simulink model "dspace_2019"  (R2019b)
settings: Solver=FixedStepDiscrete  StartTime=0.0  StopTime=Inf  FixedStep=1e-3  RelTol=1e-3
PostLoadFcn:
  | , if any(exist('dsrtsu_mdlpostloadfcn', 'file') ~= 0), dsrtsu_mdlpostloadfcn('Execute', bdroot); end,
undefined symbols (not defined in the file): ami, amk1_setpoints_1, amk2_setpoints_1, amk3_setpoints_1, amk4_setpoints_1, as, digital, ebs, indicator, mcu_set_dbu_indicator_points, mcu_set_ecu_indicator_points, res_ntm_node_control
libraries: rtican x63, simulink x5, rti1401lib_dio_type3 x4, simulink_extras x1
(part 16 of 16)

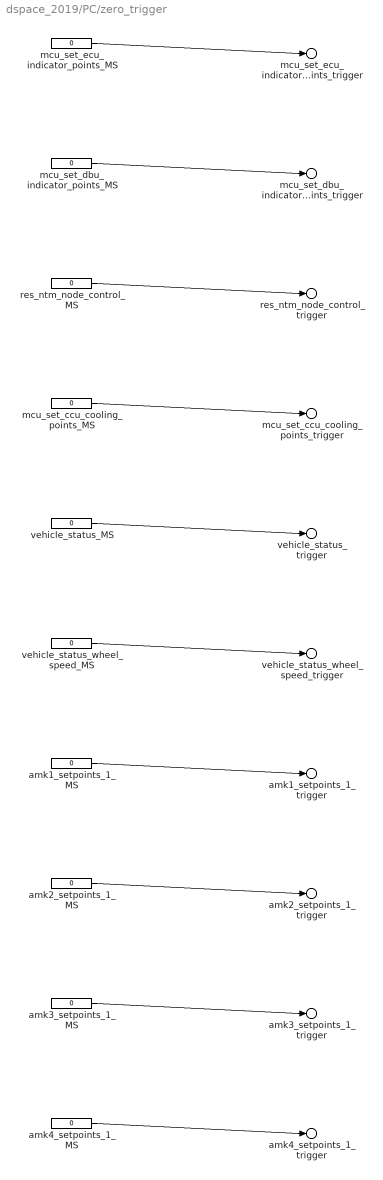
== system dspace_2019/PC/zero_trigger ==
  amk1_setpoints_1_MS : Constant  Value=0
  amk2_setpoints_1_MS : Constant  Value=0
  amk3_setpoints_1_MS : Constant  Value=0
  amk4_setpoints_1_MS : Constant  Value=0
  mcu_set_ccu_cooling_points_MS : Constant  Value=0
  mcu_set_dbu_indicator_points_MS : Constant  Value=0
  mcu_set_ecu_indicator_points_MS : Constant  Value=0
  res_ntm_node_control_MS : Constant  Value=0
  vehicle_status_MS : Constant  Value=0
  vehicle_status_wheel_speed_MS : Constant  Value=0
  mcu_set_ecu_indicator_points_trigger : Outport  PortName=triggers  Element=mcu_set_ecu_indicator_points
  mcu_set_dbu_indicator_points_trigger : Outport  PortName=triggers  Element=mcu_set_dbu_indicator_points
  res_ntm_node_control_trigger : Outport  PortName=triggers  Element=res_ntm_node_control
  mcu_set_ccu_cooling_points_trigger : Outport  PortName=triggers  Element=mcu_set_ccu_cooling_points
  vehicle_status_trigger : Outport  PortName=triggers  Element=vehicle_status
  vehicle_status_wheel_speed_trigger : Outport  PortName=triggers  Element=vehicle_status_wheel_speed
  amk1_setpoints_1_trigger : Outport  PortName=triggers  Element=amk1_setpoints_1
  amk2_setpoints_1_trigger : Outport  PortName=triggers  Element=amk2_setpoints_1
  amk3_setpoints_1_trigger : Outport  PortName=triggers  Element=amk3_setpoints_1
  amk4_setpoints_1_trigger : Outport  PortName=triggers  Element=amk4_setpoints_1
  wires:
  mcu_set_ecu_indicator_points_MS/1 -> mcu_set_ecu_indicator_points_trigger/1
  mcu_set_dbu_indicator_points_MS/1 -> mcu_set_dbu_indicator_points_trigger/1
  res_ntm_node_control_MS/1 -> res_ntm_node_control_trigger/1
  mcu_set_ccu_cooling_points_MS/1 -> mcu_set_ccu_cooling_points_trigger/1
  vehicle_status_MS/1 -> vehicle_status_trigger/1
  vehicle_status_wheel_speed_MS/1 -> vehicle_status_wheel_speed_trigger/1
  amk1_setpoints_1_MS/1 -> amk1_setpoints_1_trigger/1
  amk2_setpoints_1_MS/1 -> amk2_setpoints_1_trigger/1
  amk3_setpoints_1_MS/1 -> amk3_setpoints_1_trigger/1
  amk4_setpoints_1_MS/1 -> amk4_setpoints_1_trigger/1

== system dspace_2019/PC/zero_tx  ==
  inner : Subsystem
  mcu_set_ecu_indicator_points_outbus : Outport  PortName=signals  Element=mcu_set_ecu_indicator_points
  mcu_set_dbu_indicator_points_outbus : Outport  PortName=signals  Element=mcu_set_dbu_indicator_points
  res_ntm_node_control_outbus : Outport  PortName=signals  Element=res_ntm_node_control
  mcu_set_ccu_cooling_points_outbus : Outport  PortName=signals  Element=mcu_set_ccu_cooling_points
  vehicle_status_outbus : Outport  PortName=signals  Element=vehicle_status
  vehicle_status_wheel_speed_outbus : Outport  PortName=signals  Element=vehicle_status_wheel_speed
  amk1_setpoints_1_outbus : Outport  PortName=signals  Element=amk1_setpoints_1
  amk2_setpoints_1_outbus : Outport  PortName=signals  Element=amk2_setpoints_1
  amk3_setpoints_1_outbus : Outport  PortName=signals  Element=amk3_setpoints_1
  amk4_setpoints_1_outbus : Outport  PortName=signals  Element=amk4_setpoints_1
  wires:
  inner/10(mcu_set_ecu_indicator_points) -> mcu_set_ecu_indicator_points_outbus/1
  inner/9(mcu_set_dbu_indicator_points) -> mcu_set_dbu_indicator_points_outbus/1
  inner/8(res_ntm_node_control) -> res_ntm_node_control_outbus/1
  inner/7(mcu_set_ccu_cooling_points) -> mcu_set_ccu_cooling_points_outbus/1
  inner/6(vehicle_status) -> vehicle_status_outbus/1
  inner/5(vehicle_status_wheel_speed) -> vehicle_status_wheel_speed_outbus/1
  inner/4(amk1_setpoints_1) -> amk1_setpoints_1_outbus/1
  inner/3(amk2_setpoints_1) -> amk2_setpoints_1_outbus/1
  inner/2(amk3_setpoints_1) -> amk3_setpoints_1_outbus/1
  inner/1(amk4_setpoints_1) -> amk4_setpoints_1_outbus/1

== system dspace_2019/RTI Data/RTI Data Store ==
  RTI Data Store : Subsystem  mask(RTI_DATA_STORE){}
      mask help:
      | RTI Data Store Block. This block is used by RTI to store internal model dependent data. Deleting this block will result in data loss.
      |
      | NEVER DELETE, COPY, OR MODIFY THIS BLOCK!
      mask Help:
      | RTI Data Store Block. This block is used by RTI to store internal model dependent data. Deleting this block will result in data loss.
      | 
      | NEVER DELETE, COPY, OR MODIFY THIS BLOCK!
      mask Display: text(0.5, 0.5, ' ', 'HorizontalAlignment', 'center');

== system dspace_2019/PC/plausability_check/implausability_logic ==
  apps1 : Inport
  apps2 : Inport  Port=2
  Compare To Constant : simulink/Logic and Bit Operations/Compare To Constant  relop=>  const=0.1  OutDataTypeStr=boolean
  Integrator : Integrator  ExternalReset=falling
  MATLAB Function2 : MATLAB Function  TreatAsAtomicUnit=on
  implausability : Outport
  wires:
  apps2/1 -> MATLAB Function2/2(apps2)
  apps1/1 -> MATLAB Function2/1(apps1)
  Compare To Constant/1 -> implausability/1
  MATLAB Function2/1(implausability) -> Integrator/2, Integrator/1
  Integrator/1 -> Compare To Constant/1

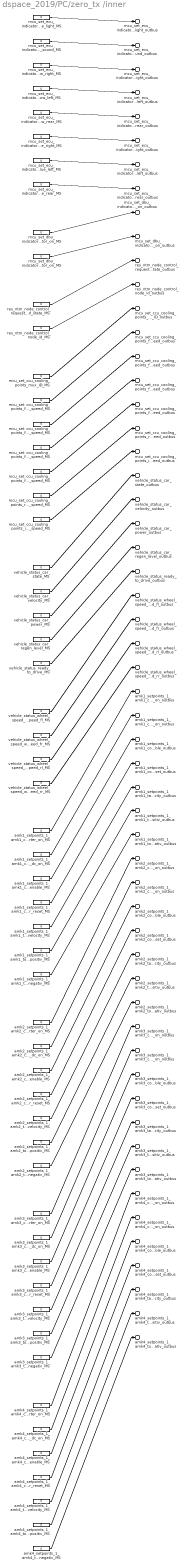
== system dspace_2019/PC/zero_tx /inner ==
  amk1_setpoints_1_amk1_control_dc_on_MS : Constant  Value=0
  amk1_setpoints_1_amk1_control_enable_MS : Constant  Value=0
  amk1_setpoints_1_amk1_control_error_reset_MS : Constant  Value=0
  amk1_setpoints_1_amk1_control_inverter_on_MS : Constant  Value=0
  amk1_setpoints_1_amk1_target_velocity_MS : Constant  Value=0
  amk1_setpoints_1_amk1_torque_limit_negativ_MS : Constant  Value=0
  amk1_setpoints_1_amk1_torque_limit_positiv_MS : Constant  Value=0
  amk2_setpoints_1_amk2_control_dc_on_MS : Constant  Value=0
  amk2_setpoints_1_amk2_control_enable_MS : Constant  Value=0
  amk2_setpoints_1_amk2_control_error_reset_MS : Constant  Value=0
  amk2_setpoints_1_amk2_control_inverter_on_MS : Constant  Value=0
  amk2_setpoints_1_amk2_target_velocity_MS : Constant  Value=0
  amk2_setpoints_1_amk2_torque_limit_negativ_MS : Constant  Value=0
  amk2_setpoints_1_amk2_torque_limit_positiv_MS : Constant  Value=0
  amk3_setpoints_1_amk3_control_dc_on_MS : Constant  Value=0
  amk3_setpoints_1_amk3_control_enable_MS : Constant  Value=0
  amk3_setpoints_1_amk3_control_error_reset_MS : Constant  Value=0
  amk3_setpoints_1_amk3_control_inverter_on_MS : Constant  Value=0
  amk3_setpoints_1_amk3_target_velocity_MS : Constant  Value=0
  amk3_setpoints_1_amk3_torque_limit_negativ_MS : Constant  Value=0
  amk3_setpoints_1_amk3_torque_limit_positiv_MS : Constant  Value=0
  amk4_setpoints_1_amk4_control_dc_on_MS : Constant  Value=0
  amk4_setpoints_1_amk4_control_enable_MS : Constant  Value=0
  amk4_setpoints_1_amk4_control_error_reset_MS : Constant  Value=0
  amk4_setpoints_1_amk4_control_inverter_on_MS : Constant  Value=0
  amk4_setpoints_1_amk4_target_velocity_MS : Constant  Value=0
  amk4_setpoints_1_amk4_torque_limit_negativ_MS : Constant  Value=0
  amk4_setpoints_1_amk4_torque_limit_positiv_MS : Constant  Value=0
  mcu_set_ccu_cooling_points_fan1_speed_MS : Constant  Value=0
  mcu_set_ccu_cooling_points_fan2_speed_MS : Constant  Value=0
  mcu_set_ccu_cooling_points_fan3_speed_MS : Constant  Value=0
  mcu_set_ccu_cooling_points_fron_pump_speed_MS : Constant  Value=0
  mcu_set_ccu_cooling_points_inverter_pump_speed_MS : Constant  Value=0
  mcu_set_ccu_cooling_points_mux_ID_MS : Constant  Value=0
  mcu_set_ccu_cooling_points_rear_pump_speed_MS : Constant  Value=0
  mcu_set_dbu_indicator_points_r2d_indicator_on_MS : Constant  Value=0
  mcu_set_dbu_indicator_points_ts_indicator_on_MS : Constant  Value=0
  mcu_set_ecu_indicator_points_assi_blue_left_MS : Constant  Value=0
  mcu_set_ecu_indicator_points_assi_blue_rear_MS : Constant  Value=0
  mcu_set_ecu_indicator_points_assi_blue_right_MS : Constant  Value=0
  mcu_set_ecu_indicator_points_assi_yellow_left_MS : Constant  Value=0
  mcu_set_ecu_indicator_points_assi_yellow_rear_MS : Constant  Value=0
  mcu_set_ecu_indicator_points_assi_yellow_right_MS : Constant  Value=0
  mcu_set_ecu_indicator_points_brake_light_MS : Constant  Value=0
  mcu_set_ecu_indicator_points_r2d_sound_MS : Constant  Value=0
  res_ntm_node_control_node_id_MS : Constant  Value=0
  res_ntm_node_control_requested_state_MS : Constant  Value=0
  vehicle_status_car_power_MS : Constant  Value=0
  vehicle_status_car_regen_level_MS : Constant  Value=0
  vehicle_status_car_state_MS : Constant  Value=0
  vehicle_status_car_velocity_MS : Constant  Value=0
  vehicle_status_ready_to_drive_MS : Constant  Value=0
  vehicle_status_wheel_speed_wheel_speed_fl_MS : Constant  Value=0
  vehicle_status_wheel_speed_wheel_speed_fr_MS : Constant  Value=0
  vehicle_status_wheel_speed_wheel_speed_rl_MS : Constant  Value=0
  vehicle_status_wheel_speed_wheel_speed_rr_MS : Constant  Value=0
  amk4_setpoints_1_amk4_control_inverter_on_outbus : Outport  PortName=amk4_setpoints_1  Element=amk4_control_inverter_on
  amk4_setpoints_1_amk4_control_dc_on_outbus : Outport  PortName=amk4_setpoints_1  Element=amk4_control_dc_on
  amk4_setpoints_1_amk4_control_enable_outbus : Outport  PortName=amk4_setpoints_1  Element=amk4_control_enable
  amk4_setpoints_1_amk4_control_error_reset_outbus : Outport  PortName=amk4_setpoints_1  Element=amk4_control_error_reset
  amk4_setpoints_1_amk4_target_velocity_outbus : Outport  PortName=amk4_setpoints_1  Element=amk4_target_velocity
  amk4_setpoints_1_amk4_torque_limit_positiv_outbus : Outport  PortName=amk4_setpoints_1  Element=amk4_torque_limit_positiv
  amk4_setpoints_1_amk4_torque_limit_negativ_outbus : Outport  PortName=amk4_setpoints_1  Element=amk4_torque_limit_negativ
  amk3_setpoints_1_amk3_control_inverter_on_outbus : Outport  Port=2  PortName=amk3_setpoints_1  Element=amk3_control_inverter_on
  amk3_setpoints_1_amk3_control_dc_on_outbus : Outport  Port=2  PortName=amk3_setpoints_1  Element=amk3_control_dc_on
  amk3_setpoints_1_amk3_control_enable_outbus : Outport  Port=2  PortName=amk3_setpoints_1  Element=amk3_control_enable
  amk3_setpoints_1_amk3_control_error_reset_outbus : Outport  Port=2  PortName=amk3_setpoints_1  Element=amk3_control_error_reset
  amk3_setpoints_1_amk3_target_velocity_outbus : Outport  Port=2  PortName=amk3_setpoints_1  Element=amk3_target_velocity
  amk3_setpoints_1_amk3_torque_limit_positiv_outbus : Outport  Port=2  PortName=amk3_setpoints_1  Element=amk3_torque_limit_positiv
  amk3_setpoints_1_amk3_torque_limit_negativ_outbus : Outport  Port=2  PortName=amk3_setpoints_1  Element=amk3_torque_limit_negativ
  amk2_setpoints_1_amk2_control_inverter_on_outbus : Outport  Port=3  PortName=amk2_setpoints_1  Element=amk2_control_inverter_on
  amk2_setpoints_1_amk2_control_dc_on_outbus : Outport  Port=3  PortName=amk2_setpoints_1  Element=amk2_control_dc_on
  amk2_setpoints_1_amk2_control_enable_outbus : Outport  Port=3  PortName=amk2_setpoints_1  Element=amk2_control_enable
  amk2_setpoints_1_amk2_control_error_reset_outbus : Outport  Port=3  PortName=amk2_setpoints_1  Element=amk2_control_error_reset
  amk2_setpoints_1_amk2_target_velocity_outbus : Outport  Port=3  PortName=amk2_setpoints_1  Element=amk2_target_velocity
  amk2_setpoints_1_amk2_torque_limit_positiv_outbus : Outport  Port=3  PortName=amk2_setpoints_1  Element=amk2_torque_limit_positiv
  amk2_setpoints_1_amk2_torque_limit_negativ_outbus : Outport  Port=3  PortName=amk2_setpoints_1  Element=amk2_torque_limit_negativ
  amk1_setpoints_1_amk1_control_inverter_on_outbus : Outport  Port=4  PortName=amk1_setpoints_1  Element=amk1_control_inverter_on
  amk1_setpoints_1_amk1_control_dc_on_outbus : Outport  Port=4  PortName=amk1_setpoints_1  Element=amk1_control_dc_on
  amk1_setpoints_1_amk1_control_enable_outbus : Outport  Port=4  PortName=amk1_setpoints_1  Element=amk1_control_enable
  amk1_setpoints_1_amk1_control_error_reset_outbus : Outport  Port=4  PortName=amk1_setpoints_1  Element=amk1_control_error_reset
  amk1_setpoints_1_amk1_target_velocity_outbus : Outport  Port=4  PortName=amk1_setpoints_1  Element=amk1_target_velocity
  amk1_setpoints_1_amk1_torque_limit_positiv_outbus : Outport  Port=4  PortName=amk1_setpoints_1  Element=amk1_torque_limit_positiv
  amk1_setpoints_1_amk1_torque_limit_negativ_outbus : Outport  Port=4  PortName=amk1_setpoints_1  Element=amk1_torque_limit_negativ
  vehicle_status_wheel_speed_wheel_speed_fl_outbus : Outport  Port=5  PortName=vehicle_status_wheel_speed  Element=wheel_speed_fl
  vehicle_status_wheel_speed_wheel_speed_fr_outbus : Outport  Port=5  PortName=vehicle_status_wheel_speed  Element=wheel_speed_fr
  vehicle_status_wheel_speed_wheel_speed_rl_outbus : Outport  Port=5  PortName=vehicle_status_wheel_speed  Element=wheel_speed_rl
  vehicle_status_wheel_speed_wheel_speed_rr_outbus : Outport  Port=5  PortName=vehicle_status_wheel_speed  Element=wheel_speed_rr
  vehicle_status_car_state_outbus : Outport  Port=6  PortName=vehicle_status  Element=car_state
  vehicle_status_car_velocity_outbus : Outport  Port=6  PortName=vehicle_status  Element=car_velocity
  vehicle_status_car_power_outbus : Outport  Port=6  PortName=vehicle_status  Element=car_power
  vehicle_status_car_regen_level_outbus : Outport  Port=6  PortName=vehicle_status  Element=car_regen_level
  vehicle_status_ready_to_drive_outbus : Outport  Port=6  PortName=vehicle_status  Element=ready_to_drive
  mcu_set_ccu_cooling_points_mux_ID_outbus : Outport  Port=7  PortName=mcu_set_ccu_cooling_points  Element=mux_ID
  mcu_set_ccu_cooling_points_fan1_speed_outbus : Outport  Port=7  PortName=mcu_set_ccu_cooling_points  Element=fan1_speed
  mcu_set_ccu_cooling_points_fan2_speed_outbus : Outport  Port=7  PortName=mcu_set_ccu_cooling_points  Element=fan2_speed
  mcu_set_ccu_cooling_points_fan3_speed_outbus : Outport  Port=7  PortName=mcu_set_ccu_cooling_points  Element=fan3_speed
  mcu_set_ccu_cooling_points_fron_pump_speed_outbus : Outport  Port=7  PortName=mcu_set_ccu_cooling_points  Element=fron_pump_speed
  mcu_set_ccu_cooling_points_rear_pump_speed_outbus : Outport  Port=7  PortName=mcu_set_ccu_cooling_points  Element=rear_pump_speed
  mcu_set_ccu_cooling_points_inverter_pump_speed_outbus : Outport  Port=7  PortName=mcu_set_ccu_cooling_points  Element=inverter_pump_speed
  res_ntm_node_control_requested_state_outbus : Outport  Port=8  PortName=res_ntm_node_control  Element=requested_state
  res_ntm_node_control_node_id_outbus : Outport  Port=8  PortName=res_ntm_node_control  Element=node_id
  mcu_set_dbu_indicator_points_ts_indicator_on_outbus : Outport  Port=9  PortName=mcu_set_dbu_indicator_points  Element=ts_indicator_on
  mcu_set_dbu_indicator_points_r2d_indicator_on_outbus : Outport  Port=9  PortName=mcu_set_dbu_indicator_points  Element=r2d_indicator_on
  mcu_set_ecu_indicator_points_brake_light_outbus : Outport  Port=10  PortName=mcu_set_ecu_indicator_points  Element=brake_light
  mcu_set_ecu_indicator_points_r2d_sound_outbus : Outport  Port=10  PortName=mcu_set_ecu_indicator_points  Element=r2d_sound
  mcu_set_ecu_indicator_points_assi_yellow_right_outbus : Outport  Port=10  PortName=mcu_set_ecu_indicator_points  Element=assi_yellow_right
  mcu_set_ecu_indicator_points_assi_yellow_left_outbus : Outport  Port=10  PortName=mcu_set_ecu_indicator_points  Element=assi_yellow_left
  mcu_set_ecu_indicator_points_assi_yellow_rear_outbus : Outport  Port=10  PortName=mcu_set_ecu_indicator_points  Element=assi_yellow_rear
  mcu_set_ecu_indicator_points_assi_blue_right_outbus : Outport  Port=10  PortName=mcu_set_ecu_indicator_points  Element=assi_blue_right
  mcu_set_ecu_indicator_points_assi_blue_left_outbus : Outport  Port=10  PortName=mcu_set_ecu_indicator_points  Element=assi_blue_left
  mcu_set_ecu_indicator_points_assi_blue_rear_outbus : Outport  Port=10  PortName=mcu_set_ecu_indicator_points  Element=assi_blue_rear
  wires:
  mcu_set_ecu_indicator_points_brake_light_MS/1 -> mcu_set_ecu_indicator_points_brake_light_outbus/1
  mcu_set_ecu_indicator_points_r2d_sound_MS/1 -> mcu_set_ecu_indicator_points_r2d_sound_outbus/1
  mcu_set_ecu_indicator_points_assi_yellow_right_MS/1 -> mcu_set_ecu_indicator_points_assi_yellow_right_outbus/1
  mcu_set_ecu_indicator_points_assi_yellow_left_MS/1 -> mcu_set_ecu_indicator_points_assi_yellow_left_outbus/1
  mcu_set_ecu_indicator_points_assi_yellow_rear_MS/1 -> mcu_set_ecu_indicator_points_assi_yellow_rear_outbus/1
  mcu_set_ecu_indicator_points_assi_blue_right_MS/1 -> mcu_set_ecu_indicator_points_assi_blue_right_outbus/1
  mcu_set_ecu_indicator_points_assi_blue_left_MS/1 -> mcu_set_ecu_indicator_points_assi_blue_left_outbus/1
  mcu_set_ecu_indicator_points_assi_blue_rear_MS/1 -> mcu_set_ecu_indicator_points_assi_blue_rear_outbus/1
  mcu_set_dbu_indicator_points_ts_indicator_on_MS/1 -> mcu_set_dbu_indicator_points_ts_indicator_on_outbus/1
  mcu_set_dbu_indicator_points_r2d_indicator_on_MS/1 -> mcu_set_dbu_indicator_points_r2d_indicator_on_outbus/1
  res_ntm_node_control_requested_state_MS/1 -> res_ntm_node_control_requested_state_outbus/1
  res_ntm_node_control_node_id_MS/1 -> res_ntm_node_control_node_id_outbus/1
  mcu_set_ccu_cooling_points_mux_ID_MS/1 -> mcu_set_ccu_cooling_points_mux_ID_outbus/1
  mcu_set_ccu_cooling_points_fan1_speed_MS/1 -> mcu_set_ccu_cooling_points_fan1_speed_outbus/1
  mcu_set_ccu_cooling_points_fan2_speed_MS/1 -> mcu_set_ccu_cooling_points_fan2_speed_outbus/1
  mcu_set_ccu_cooling_points_fan3_speed_MS/1 -> mcu_set_ccu_cooling_points_fan3_speed_outbus/1
  mcu_set_ccu_cooling_points_fron_pump_speed_MS/1 -> mcu_set_ccu_cooling_points_fron_pump_speed_outbus/1
  mcu_set_ccu_cooling_points_rear_pump_speed_MS/1 -> mcu_set_ccu_cooling_points_rear_pump_speed_outbus/1
  mcu_set_ccu_cooling_points_inverter_pump_speed_MS/1 -> mcu_set_ccu_cooling_points_inverter_pump_speed_outbus/1
  vehicle_status_car_state_MS/1 -> vehicle_status_car_state_outbus/1
  vehicle_status_car_velocity_MS/1 -> vehicle_status_car_velocity_outbus/1
  vehicle_status_car_power_MS/1 -> vehicle_status_car_power_outbus/1
  vehicle_status_car_regen_level_MS/1 -> vehicle_status_car_regen_level_outbus/1
  vehicle_status_ready_to_drive_MS/1 -> vehicle_status_ready_to_drive_outbus/1
  vehicle_status_wheel_speed_wheel_speed_fl_MS/1 -> vehicle_status_wheel_speed_wheel_speed_fl_outbus/1
  vehicle_status_wheel_speed_wheel_speed_fr_MS/1 -> vehicle_status_wheel_speed_wheel_speed_fr_outbus/1
  vehicle_status_wheel_speed_wheel_speed_rl_MS/1 -> vehicle_status_wheel_speed_wheel_speed_rl_outbus/1
  vehicle_status_wheel_speed_wheel_speed_rr_MS/1 -> vehicle_status_wheel_speed_wheel_speed_rr_outbus/1
  amk1_setpoints_1_amk1_control_inverter_on_MS/1 -> amk1_setpoints_1_amk1_control_inverter_on_outbus/1
  amk1_setpoints_1_amk1_control_dc_on_MS/1 -> amk1_setpoints_1_amk1_control_dc_on_outbus/1
  amk1_setpoints_1_amk1_control_enable_MS/1 -> amk1_setpoints_1_amk1_control_enable_outbus/1
  amk1_setpoints_1_amk1_control_error_reset_MS/1 -> amk1_setpoints_1_amk1_control_error_reset_outbus/1
  amk1_setpoints_1_amk1_target_velocity_MS/1 -> amk1_setpoints_1_amk1_target_velocity_outbus/1
  amk1_setpoints_1_amk1_torque_limit_positiv_MS/1 -> amk1_setpoints_1_amk1_torque_limit_positiv_outbus/1
  amk1_setpoints_1_amk1_torque_limit_negativ_MS/1 -> amk1_setpoints_1_amk1_torque_limit_negativ_outbus/1
  amk2_setpoints_1_amk2_control_inverter_on_MS/1 -> amk2_setpoints_1_amk2_control_inverter_on_outbus/1
  amk2_setpoints_1_amk2_control_dc_on_MS/1 -> amk2_setpoints_1_amk2_control_dc_on_outbus/1
  amk2_setpoints_1_amk2_control_enable_MS/1 -> amk2_setpoints_1_amk2_control_enable_outbus/1
  amk2_setpoints_1_amk2_control_error_reset_MS/1 -> amk2_setpoints_1_amk2_control_error_reset_outbus/1
  amk2_setpoints_1_amk2_target_velocity_MS/1 -> amk2_setpoints_1_amk2_target_velocity_outbus/1
  amk2_setpoints_1_amk2_torque_limit_positiv_MS/1 -> amk2_setpoints_1_amk2_torque_limit_positiv_outbus/1
  amk2_setpoints_1_amk2_torque_limit_negativ_MS/1 -> amk2_setpoints_1_amk2_torque_limit_negativ_outbus/1
  amk3_setpoints_1_amk3_control_inverter_on_MS/1 -> amk3_setpoints_1_amk3_control_inverter_on_outbus/1
  amk3_setpoints_1_amk3_control_dc_on_MS/1 -> amk3_setpoints_1_amk3_control_dc_on_outbus/1
  amk3_setpoints_1_amk3_control_enable_MS/1 -> amk3_setpoints_1_amk3_control_enable_outbus/1
  amk3_setpoints_1_amk3_control_error_reset_MS/1 -> amk3_setpoints_1_amk3_control_error_reset_outbus/1
  amk3_setpoints_1_amk3_target_velocity_MS/1 -> amk3_setpoints_1_amk3_target_velocity_outbus/1
  amk3_setpoints_1_amk3_torque_limit_positiv_MS/1 -> amk3_setpoints_1_amk3_torque_limit_positiv_outbus/1
  amk3_setpoints_1_amk3_torque_limit_negativ_MS/1 -> amk3_setpoints_1_amk3_torque_limit_negativ_outbus/1
  amk4_setpoints_1_amk4_control_inverter_on_MS/1 -> amk4_setpoints_1_amk4_control_inverter_on_outbus/1
  amk4_setpoints_1_amk4_control_dc_on_MS/1 -> amk4_setpoints_1_amk4_control_dc_on_outbus/1
  amk4_setpoints_1_amk4_control_enable_MS/1 -> amk4_setpoints_1_amk4_control_enable_outbus/1
  amk4_setpoints_1_amk4_control_error_reset_MS/1 -> amk4_setpoints_1_amk4_control_error_reset_outbus/1
  amk4_setpoints_1_amk4_target_velocity_MS/1 -> amk4_setpoints_1_amk4_target_velocity_outbus/1
  amk4_setpoints_1_amk4_torque_limit_positiv_MS/1 -> amk4_setpoints_1_amk4_torque_limit_positiv_outbus/1
  amk4_setpoints_1_amk4_torque_limit_negativ_MS/1 -> amk4_setpoints_1_amk4_torque_limit_negativ_outbus/1

== system dspace_2019/RTI Data/RTI Data Store/RTI Data Store ==
  RTI Data Store : Subsystem  mask(RTI_DATA_STORE){}
      mask help:
      | RTI Data Store Block. This block is used by RTI to store internal model dependent data. Deleting this block will result in data loss.
      |
      | NEVER DELETE, COPY, OR MODIFY THIS BLOCK!
      mask Help:
      | RTI Data Store Block. This block is used by RTI to store internal model dependent data. Deleting this block will result in data loss.
      | 
      | NEVER DELETE, COPY, OR MODIFY THIS BLOCK!
      mask Display: text(0.5, 0.5, ' ', 'HorizontalAlignment', 'center');

== system dspace_2019/RTI Data/RTI Data Store/RTI Data Store/RTI Data Store ==
  RTI Data Store : Subsystem  mask(RTI_DATA_STORE){}
      mask help:
      | RTI Data Store Block. This block is used by RTI to store internal model dependent data. Deleting this block will result in data loss.
      |
      | NEVER DELETE, COPY, OR MODIFY THIS BLOCK!
      mask Help:
      | RTI Data Store Block. This block is used by RTI to store internal model dependent data. Deleting this block will result in data loss.
      | 
      | NEVER DELETE, COPY, OR MODIFY THIS BLOCK!
      mask Display: text(0.5, 0.5, ' ', 'HorizontalAlignment', 'center');

== system dspace_2019/RTI Data/RTI Data Store/RTI Data Store/RTI Data Store/RTI Data Store ==

== matlab function dspace_2019/Signal Preconditioning/MATLAB Function1 ==
  data: bpps1 input; normalized_brake_pedal_travel output; bpps2 input; normalized_brake_pedal_diff output
function [normalized_brake_pedal_travel, normalized_brake_pedal_diff] = fcn(bpps1, bpps2)

normalized_brake_pedal_travel_1 = (bpps1 - 1106) / (1480 - 1106);
normalized_brake_pedal_travel_2 = (bpps2 - 1024) / (1389 - 1024);

normalized_brake_pedal_diff = abs(normalized_brake_pedal_travel_2 - normalized_brake_pedal_travel_1);
normalized_brake_pedal_travel = (normalized_brake_pedal_travel_1 + normalized_brake_pedal_travel_2)/2;

== matlab function dspace_2019/Signal Preconditioning/MATLAB Function2 ==
  data: apps1 input; normalized_accelerator_pedal_travel output; apps2 input; implausability output
function [normalized_accelerator_pedal_travel, implausability] = fcn(apps1, apps2)
acc_1_min = 803;
acc_2_min = 757;
acc_1_max = 2062;
acc_2_max = 1975;

% normalized so max value = 100
normalized_accelerator_pedal_travel_1 = (apps1 - acc_1_min) / (acc_1_max - acc_1_min);
normalized_accelerator_pedal_travel_2 = (apps2 - acc_2_min) / (acc_2_max - acc_2_min);




acc_1_norm = (apps1-acc1_min)/((acc_1_max-acc_1_min)/1000); % normalized so max value = 1000
acc_2_norm = (apps2-acc_2_min)/((acc_2_max-acc_2_min)/1000);
diff = acc_1_norm-acc_2_norm;

if (abs(diff)>100) % if difference larger than 10 percentage points, implausability = true (1000 is 100.0%, 100 is 10,0%
    implausability = true;

else
    implausability = false;

end


normalized_accelerator_pedal_travel = (normalized_accelerator_pedal_travel_1 + normalized_accelerator_pedal_travel_2)/2;

% What about failure according to T11.9?

== stateflow chart dspace_2019/PC/Chart ==
  state SETUP_
  state AS_OFF_
    r2d_indicator = indicator.off;
    tsa_indicator = indicator.blinking;
    inverters = digital.inactive;
  state MANUAL_READY_
    r2d_indicator = indicator.blinking;
    tsa_indicator = indicator.continuous;
    inverters = digital.inactive;
  state MANUAL_DRIVING_
    r2d_indicator = indicator.continuous;
    r2d_buzzer = double(before(0.2, sec));
    inverters = digital.active;
  (default) -> SETUP_
  SETUP_ -> AS_OFF_
  MANUAL_READY_ -> AS_OFF_ [order 1] : [~ts_activated]
  AS_OFF_ -> MANUAL_READY_ : [(ami_state == ami.manual_driving) && (ebs_state == ebs.unavailable) && (as_state == as.off) && ts_activated]
  MANUAL_READY_ -> MANUAL_DRIVING_ [order 2] : [r2d_button && (abs(steering_angle) < 5) && (abs(accelerator_angle) < 0.1) && (abs(brake_angle) < 0.1) && after(3, sec)]
  MANUAL_DRIVING_ -> MANUAL_READY_ : [(r2d_button && (abs(vehicle_speed) < 0.1)) || (~ts_activated)]
  data: inverters output; ts_activated input; ts_off input; r2d_button input; steering_angle input; accelerator_angle input; brake_angle input; vehicle_speed input; r2d_indicator output; digital parameter; indicator parameter; ami parameter; as parameter; as_state input; ebs parameter; ebs_state input; ami_state input; tsa_indicator output; r2d_buzzer output

== matlab function dspace_2019/PC/MATLAB Function ==
  data: v1 input; y output; v2 input; v3 input; v4 input
function y = average(v1, v2, v3, v4)

y = (v1 + v2 + v3 + v4) / 4;

== matlab function dspace_2019/PC/plausability_check/implausability_logic/MATLAB Function2 ==
  data: apps1 input; apps2 input; implausability output
function implausability = fcn(apps1, apps2)
acc_1_min = 803;
acc_2_min = 757;
acc_1_max = 2062;
acc_2_max = 1975;


acc_1_norm = 100*(apps1-acc1_min)/(acc_1_max-acc_1_min); % normalized so max value = 1000
acc_2_norm = 100*(apps2-acc_2_min)/(acc_2_max-acc_2_min);
diff = acc_1_norm-acc_2_norm;

if (abs(diff)>10) % if difference larger than 10 percentage points, implausability = true 
    implausability = true;

else
    implausability = false;

end


% What about failure according to T11.9?

== matlab function dspace_2019/Vehicular Control/MATLAB Function ==
  data: car_state input; velocity output; as_speed input; accelerator_pedal input
function velocity = convert_to_velocity(car_state, as_speed, accelerator_pedal)

velocity= 0;
